simulink model "Unit_Test_Debug"  (R2018b)
settings: Solver=FixedStepDiscrete  StartTime=0.0  StopTime=100  FixedStep=fswParams.sample_time_s  RelTol=1e-3
libraries: aerolibutil x4, MEKF_lib x1, satelliteDynamics_lib x1
settings Model: Creator=satcave1  LastModifiedBy=kylle

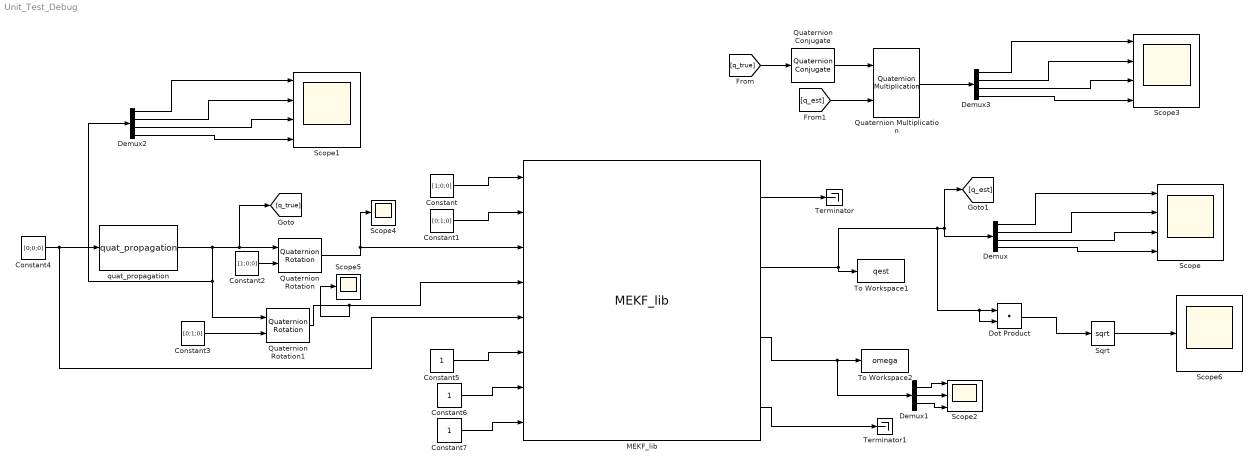
== system Unit_Test_Debug ==
  Constant : Constant  Value=[1;0;0]  VectorParams1D=off
  Constant1 : Constant  Value=[0;1;0]  VectorParams1D=off
  Constant2 : Constant  Value=[1;0;0]  VectorParams1D=off
  Constant3 : Constant  Value=[0;1;0]  VectorParams1D=off
  Constant4 : Constant  Value=[0;0;0]  VectorParams1D=off
  Constant5 : Constant
  Constant6 : Constant
  Constant7 : Constant
  Demux : Demux
  Demux1 : Demux  Outputs=3
  Demux2 : Demux
  Demux3 : Demux
  Dot Product : DotProduct  InputSameDT=on  OutDataTypeStr=Inherit: Inherit via internal rule
  MEKF_lib : MEKF_lib/MEKF_lib  SystemSampleTime=-1
  Quaternion Conjugate : aerolibutil/Quaternion Conjugate
      settings: SourceProductName=Aerospace Blockset  SourceProductBaseCode=AE
  Quaternion Multiplication : aerolibutil/Quaternion Multiplication
  Quaternion Rotation : aerolibutil/Quaternion Rotation
  Quaternion Rotation1 : aerolibutil/Quaternion Rotation
  Scope : Scope  NumInputPorts=4
  Scope1 : Scope  NumInputPorts=4
  Scope2 : Scope  NumInputPorts=3
  Scope3 : Scope  NumInputPorts=4
  Scope4 : Scope
  Scope5 : Scope
  Scope6 : Scope
  Sqrt : Sqrt  SaturateOnIntegerOverflow=on
  Terminator : Terminator
  Terminator1 : Terminator
  To Workspace1 : ToWorkspace  VariableName=qest  SaveFormat=Timeseries  SampleTime=-1
  To Workspace2 : ToWorkspace  VariableName=omega  SaveFormat=Timeseries  SampleTime=-1
  quat_propagation : satelliteDynamics_lib/satelliteDynamics_lib/quat_propagation  SystemSampleTime=-1
  wires:
  Constant/1 -> MEKF_lib/1
  Quaternion Rotation/1 -> MEKF_lib/3, Scope4/1
  Constant1/1 -> MEKF_lib/2
  Constant5/1 -> MEKF_lib/6
  Constant6/1 -> MEKF_lib/7
  Constant7/1 -> MEKF_lib/8
  MEKF_lib/1 -> Terminator/1
  MEKF_lib/2 -> To Workspace1/1, Dot Product/2, Dot Product/1, [q_est], Demux/1
  MEKF_lib/4 -> Terminator1/1
  Demux/1 -> Scope/1
  Demux/2 -> Scope/2
  Demux/3 -> Scope/3
  Demux/4 -> Scope/4
  Demux1/2 -> Scope2/2
  Demux1/1 -> Scope2/1
  Demux1/3 -> Scope2/3
  MEKF_lib/3 -> Demux1/1, To Workspace2/1
  Constant2/1 -> Quaternion Rotation/2
  Constant3/1 -> Quaternion Rotation1/2
  Constant4/1 -> MEKF_lib/5, quat_propagation/1
  Demux2/4 -> Scope1/4
  Demux2/2 -> Scope1/2
  Demux2/1 -> Scope1/1
  Demux2/3 -> Scope1/3
  quat_propagation/1 -> Demux2/1, Quaternion Rotation1/1, [q_true], Quaternion Rotation/1
  [q_true] -> Quaternion Conjugate/1
  [q_est] -> Quaternion Multiplication/2
  Quaternion Conjugate/1 -> Quaternion Multiplication/1
  Demux3/4 -> Scope3/4
  Demux3/2 -> Scope3/2
  Demux3/1 -> Scope3/1
  Demux3/3 -> Scope3/3
  Quaternion Multiplication/1 -> Demux3/1
  Quaternion Rotation1/1 -> MEKF_lib/4, Scope5/1
  Dot Product/1 -> Sqrt/1
  Sqrt/1 -> Scope6/1
